simulink model "localizeUsingLidar"  (R2021b)
settings: Solver=VariableStepAuto  StartTime=0.0  StopTime=28.964  RelTol=1e-3
PreLoadFcn:
  | data = load('ReferencePathForward.mat');
  | 
  | refPosesX = data.ReferencePathForward.refPosesX;
  | refPosesY = data.ReferencePathForward.refPosesY;
  | refPosesT = data.ReferencePathForward.refPosesT;
  | 
  | if exist('lidarLocation','var') && exist('lidarOrientation','var')
  |     initPose = [lidarLocation(1,:) lidarOrientation(1, :)];
  | else
  |     initPose = [36.0913048  -9.4484911   1.6100000           0           0  -3.1311762];
  | end
libraries: sim3dphyssensorlib x1, sim3dlib x1, sim3dautolib x1
settings Model: Creator=The MathWorks, Inc.  LastModifiedBy=The MathWorks, Inc.
settings SolverCC: AlgebraicLoopSolver=TrustRegion
settings DebuggingCC: SFMachineParentedDataDiag=warning

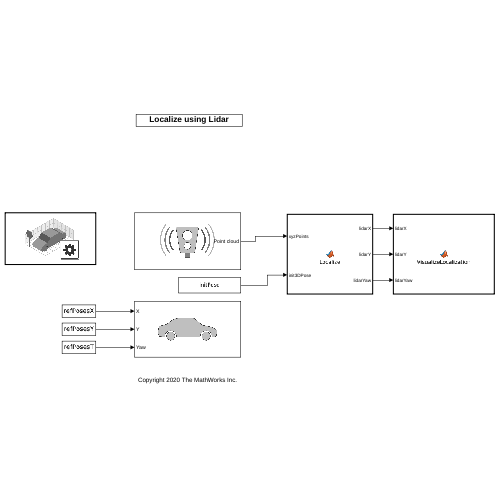
[thumbnail: Simulink's stored preview of the top-level diagram]
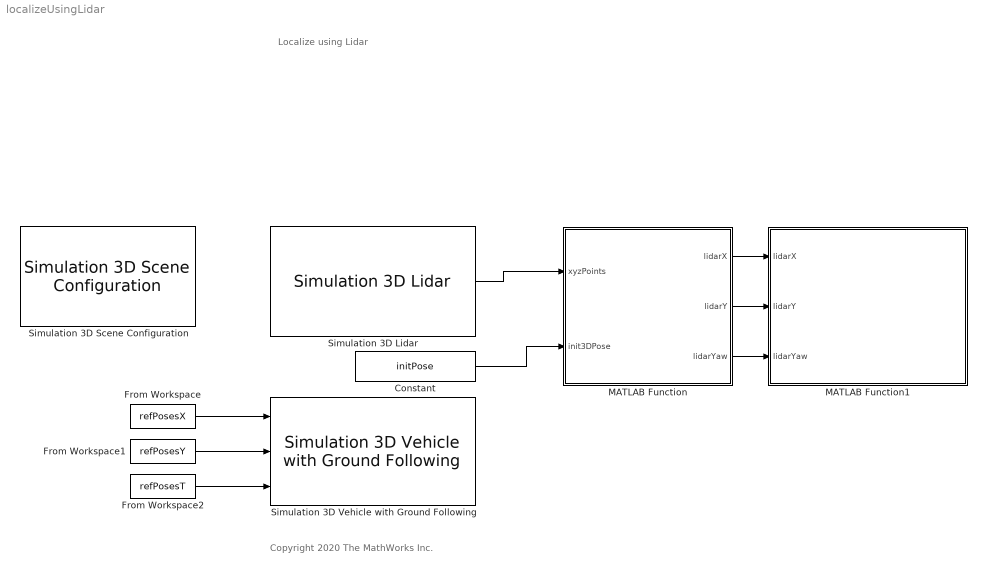
== system localizeUsingLidar ==
  note: Localize using Lidar
  note: Copyright 2020 The MathWorks Inc.
  Constant : Constant  Value=initPose  VectorParams1D=off
  From Workspace : FromWorkspace  VariableName=refPosesX  OutputAfterFinalValue=Holding final value
  From Workspace1 : FromWorkspace  VariableName=refPosesY  OutputAfterFinalValue=Holding final value
  From Workspace2 : FromWorkspace  VariableName=refPosesT  OutputAfterFinalValue=Holding final value
  MATLAB Function : MATLAB Function  TreatAsAtomicUnit=on
  MATLAB Function1 : MATLAB Function  StopFcn=|  TreatAsAtomicUnit=on
      | % Find figure by name
      | viewerFigure = findall(groot, 'type', 'figure', ...
      |     'name','Scene Map Display');
      | 
      | % Close figure
      | if ~isempty(viewerFigure)
      |     viewerFigure = viewerFigure(end);
      |     if isvalid(viewerFigure)
      |         close(viewerFigure);
      |     end
      | end
  Simulation 3D Lidar : sim3dphyssensorlib/Simulation 3D Lidar  Priority=1  sensorTag=Sim3dSensor1  sensorId=1  sensorName=Sim3dSensor1  vehTagList={'Scene Origin';'SimulinkVehicle1'}  vehTag=SimulinkVehicle1  mountLoc=Roof center  offsetFlag=off  tmountOffset=[0, 0, 0]  rmountOffset=[0, 0, 0]  DetectionRange=90  RangeResolution=0.002  VerticalFOV=40  VerticalResolution=1.25  HorizontalFOV=360  HorizontalResolution=0.332409972299169  DistanceOutportEnabled=off  TransformOutportEnabled=off  SampleTime=0.1  mountPoint=[0 0 1.55999994277954]  mountOrientation=[0 0 0]  aMode=3  ID=1
      settings: SourceProductBaseCode=AE,DR,UV,VE
  Simulation 3D Scene Configuration : sim3dlib/Simulation 3D Scene Configuration  Priority=0  ProjectFormat_internal=Default Scenes  ProjectFormat=Default Scenes  SceneDesc=Large parking lot  ProjectName=/mathworks/devel/bat/BR2021bd/build/matlab/toolbox/shared/sim3d_projects/automotive_project/UE4/LinuxNoEditor/AutoVrtlEnv.sh  ScenePath=/Game/Maps/HwStrght  vehTagList={'Scene Origin';'SimulinkVehicle1'}  vehTag=SimulinkVehicle1  OpVisEn=off  Ts=0.02  EnableWindow=on  EnableWeather=off  SunAltitude=40.0  SunAzimuth=90  clouds=10  wind=1  fog=0  rain=0  sensorTag=MainCamera2  sensorId=2  sensorName=MainCamera2  mountLoc=Origin  offsetFlag=off  tmountOffset=[0, 0, 0]  rmountOffset=[0, 0, 0]  HorizontalResolution=1280  VerticalResolution=720  HorizontalFOV=60  mountPoint=[0 0 0]  mountOrientation=[0 0 0]  aMode=3  ID=2
      settings: SourceProductBaseCode=AE,DR,UV,VE
  Simulation 3D Vehicle with Ground Following : sim3dautolib/Simulation 3D Vehicle with Ground Following  Priority=-1  PassVehMesh=Hatchback  PassVehMesh_Internal=Hatchback  MeshPath=/MathWorksSimulation/Vehicles/Muscle/Meshes/SK_MuscleCar.SK_MuscleCar  TrackWidth=1.9  WheelBase=3  WheelRadius=0.35  VehColor=Red  VehColor_Internal=Red  InitialPos=[refPosesX(1,2), refPosesY(1,2), 0]  InitialRot=[0, 0, refPosesT(1,2)]  ActorName=SimulinkVehicle1  SampleTime=0.02  ActorType=SimulinkVehicle  ID=1  aMode=3  ActorTag=SimulinkVehicle1  CoordinateScheme=ISO  VehLightsControl=off  HeadlightColor=[ 1, 1, 1 ]  HighBeamIntensity=100000  LowBeamIntensity=60000  HighBeamConeAngle=70  LowBeamConeAngle=70  LeftHeadlightOrientation=[ 0, 0 ]  RightHeadlightOrientation=[ 0, 0 ]  BrakelightIntensity=500  ReverselightIntensity=500  SignallightIntensity=500  SignallightPeriod=1  SignalPulseWidth=50  TransformOutportEnabled=off
      settings: SourceProductBaseCode=AE,DR,UV,VE
  wires:
  From Workspace2/1 -> Simulation 3D Vehicle with Ground Following/3
  From Workspace/1 -> Simulation 3D Vehicle with Ground Following/1
  From Workspace1/1 -> Simulation 3D Vehicle with Ground Following/2
  Simulation 3D Lidar/1 -> MATLAB Function/1(xyzPoints)
  MATLAB Function/1(lidarX) -> MATLAB Function1/1(lidarX)
  MATLAB Function/3(lidarYaw) -> MATLAB Function1/3(lidarYaw)
  MATLAB Function/2(lidarY) -> MATLAB Function1/2(lidarY)
  Constant/1 -> MATLAB Function/2(init3DPose)

== matlab function localizeUsingLidar/MATLAB Function ==
  data: xyzPoints input; lidarX output; lidarY output; lidarYaw output; init3DPose input
function [lidarX, lidarY, lidarYaw] = Localize(xyzPoints, init3DPose)

coder.extrinsic('pointCloud', 'helperLidarRegistrationLocalizer', ...
    'localize', 'updateDisplay', 'rigid3d', 'helperExtract2DPose', 'struct', ...
    'helperPoseToRigidTransform', 'helperInterpolatePoseTform');

persistent frameCount lidarLocalizer relPoseTform currPoseTform isLocalizerActive;

if isempty(frameCount)
    frameCount = 0;
end
if isempty(lidarLocalizer)
    % Convert the pose to a rigid transformation object
    initTform = helperPoseToRigidTransform(init3DPose);
    
    % Rigid transformation object to convert from lidar sensor frame to
    % vehicle frame. See
    % https://www.mathworks.com/help/driving/ref/hatchback.html for more
    % details.
    lidarToVehicleTform = helperPoseToRigidTransform(single([0 0 -1.57 0 0 0]));
    
    % Specify display preferences
    displayPrefs = struct(...
        'View',                 '2D', ...                   % Display 2D top-view
        'VehicleDimensions',    [3.864, 1.960, 1.286], ...  % [length, width, height] of vehicle
        'VehicleColor',         [0.85 0.325 0.098], ...     % [R, G, B] color used to display vehicle
        'PoseOffset',           [0 0 -1.57], ...            % [x, y, z] offset to add to pose 
        'Limits',               [0 50 -25 10 -30 30], ...   % [xmin, xmax, ymin, ymax, zmin, zmax] map limits
        'Location',             'west');
    
    % Create a registration-based lidar localizer
    lidarLocalizer = helperLidarRegistrationLocalizer(...
        'InitialPoseTransform',     initTform, ...
        'LidarToVehicleTransform',  lidarToVehicleTform, ...
        'DisplayPreferences',       displayPrefs);
end

if isempty(currPoseTform)
    currPoseTform = rigid3d(eye(4,'single'));
end
if isempty(relPoseTform)
    relPoseTform = rigid3d(eye(4,'single'));
end
if isempty(isLocalizerActive)
    isLocalizerActive = false;
end

frameCount = frameCount + 1;

% Ignore first two frames
% Ignore point cloud with no valid points
hasNoPoints = all( isnan(xyzPoints), 'all' );
if hasNoPoints || frameCount < 2
    lidarX   = single(NaN);
    lidarY   = single(NaN);
    lidarYaw = single(NaN);
    return;
end

skipFrames = 5;
if mod(frameCount-1, skipFrames)==0
    isLocalizerActive = true;
    ptCloud = pointCloud(xyzPoints);
    
    [currPoseTform, relPoseTform] = localize(lidarLocalizer, ptCloud);
    
    updateDisplay(lidarLocalizer);
    drawnow update
    
    currPose = helperExtract2DPose(currPoseTform);
    
    lidarX      = currPose(1);
    lidarY      = currPose(2);
    lidarYaw    = currPose(3); % in radians
else
    if ~isLocalizerActive
        lidarX   = single(NaN);
        lidarY   = single(NaN);
        lidarYaw = single(NaN);
        return;
    end
    
    % Interpolate between current pose transform and next pose transform,
    % i.e. assume constant velocity motion
    t = mod(frameCount-1, skipFrames)  / skipFrames;
    interpPoseTform = helperInterpolatePoseTform(currPoseTform, relPoseTform, t);
    
    currPose = helperExtract2DPose(interpPoseTform);
    
    lidarX   = currPose(1);
    lidarY   = currPose(2);
    lidarYaw = currPose(3);
end

end

== matlab function localizeUsingLidar/MATLAB Function1 ==
  data: lidarX input; lidarY input; lidarYaw input
function VisualizeLocalization(lidarX, lidarY, lidarYaw)
%VisualizeLocalizationPath Visualize localization path.

coder.extrinsic('helperGetSceneImage', 'figure', 'imshow', 'title', ...
    'get', 'set', 'movegui', 'gca', 'isvalid', 'hold','showShape', 'scatter', ...
    'helperUpdateScatter', 'xlim', 'ylim');

persistent hFig hAx hSc;

vehicleColor = [0.85 0.325 0.098];
vehicleDims  = [3.864 1.960];
markerSize   = 8;
if isempty(hFig)
    % Query the model to find the scene selection
    sceneName = 'LargeParkingLot';
    [sceneImage, sceneRef] = helperGetSceneImage(sceneName);
    
    % Create a figure and display the scene on it
    hFig = figure('Name', 'Scene Map Display');
    hIm = imshow(sceneImage, sceneRef, 'InitialMagnification', 12.5);
    hAx  = get(hIm,'Parent');
    set(hAx, 'YDir', 'normal');
    title(hAx, 'Localization estimate');
    xlim(hAx, [  0 50]);
    ylim(hAx, [-25 10]);
    
    hold(hAx, 'on')
    hSc = scatter(hAx, NaN, NaN, markerSize, vehicleColor, 'filled');
    hold(hAx, 'off')
    
    % Move figure to right of screen
    movegui(hFig, 'east');
end

if isvalid(hFig) && isfinite(lidarX) && isfinite(lidarY) && isfinite(lidarYaw)
    showShape('rectangle', [lidarX lidarY vehicleDims rad2deg(lidarYaw)], ...
        'Parent', hAx, 'Color', vehicleColor, 'Opacity', 0.2);
    
    helperUpdateScatter(hSc, lidarX, lidarY);
end
end
